simulink model "main"  (R2016b)
settings: Solver=VariableStepAuto  StartTime=0.0  StopTime=0.4  FixedStep=2e-4  RelTol=1e-3
values from neighbouring files (symbols this model uses):
  denGc = denGc{1}    [rigidBodyInit.m]
  numGc = numGc{1}    [rigidBodyInit.m]
  Ts = 1/fs    (= 0.0002)    [rigidBodyInit.m]
undefined symbols (not defined in the file or in its folder): denGp, denGpDis, numGp, numGpDis, TsN
libraries: model_controller x3, simulink x1
settings Model: Creator=Dai Luyao  LastModifiedBy=Dai Luyao

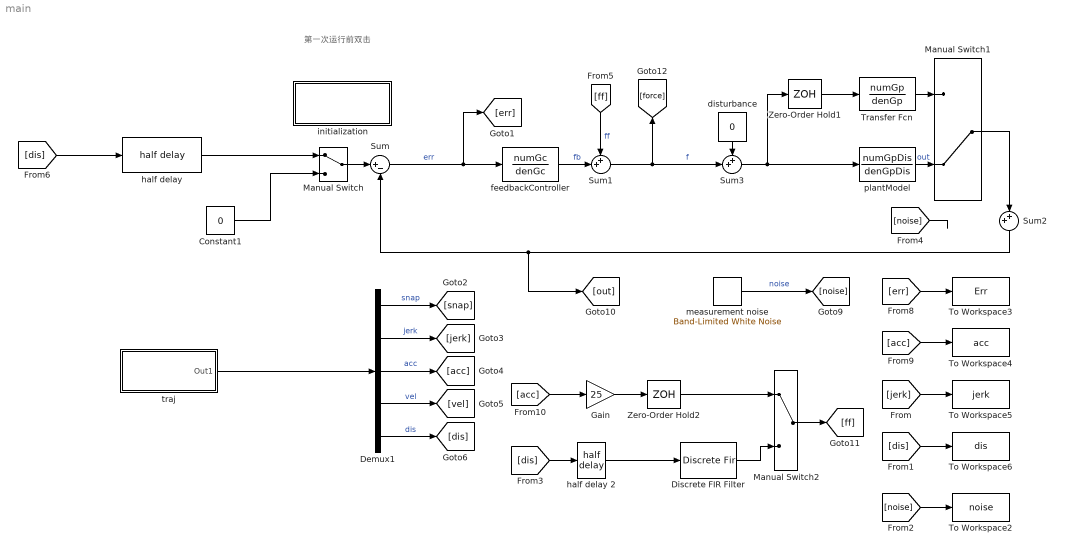
== system main ==
  note: 第一次运行前双击
  Constant1 : Constant  Value=0
  Demux1 : Demux  Outputs=5
  Discrete FIR Filter : DiscreteFir  Coefficients=denGpDis*6.25e8  SampleTime=Ts
  Gain : Gain  Gain=25
  Manual Switch : ManualSwitch
  Manual Switch1 : ManualSwitch  CurrentSetting=0
  Manual Switch2 : ManualSwitch
  Sum : Sum  Inputs=|+-
  Sum1 : Sum  Inputs=++|
  Sum2 : Sum  Inputs=++|
  Sum3 : Sum  Inputs=++|
  To Workspace2 : ToWorkspace  VariableName=noise  SaveFormat=Structure With Time  SampleTime=-1
  To Workspace3 : ToWorkspace  VariableName=Err  SaveFormat=Structure With Time  SampleTime=-1
  To Workspace4 : ToWorkspace  VariableName=acc  SaveFormat=Structure With Time  SampleTime=-1
  To Workspace5 : ToWorkspace  VariableName=jerk  SaveFormat=Structure With Time  SampleTime=-1
  To Workspace6 : ToWorkspace  VariableName=dis  SaveFormat=Structure With Time  SampleTime=-1
  Transfer Fcn : TransferFcn  Numerator=numGp  Denominator=denGp
  Zero-Order Hold1 : ZeroOrderHold  SampleTime=Ts
  Zero-Order Hold2 : ZeroOrderHold  SampleTime=Ts
  disturbance : Constant  Value=0
  feedbackController : DiscreteTransferFcn  Numerator=numGc  Denominator=denGc  SampleTime=Ts
  "half delay " : model_controller/Profile Generators/half delay 
  half delay 2 : model_controller/Profile Generators/half delay 
  initialization : Subsystem
      settings: OpenFcn=initiateSimulation;  MoveFcn=edit initiateSimulation;
  measurement noise : simulink/Sources/Band-Limited White Noise  Cov=noisePower  Ts=TsN  seed=[23341]
  plantModel : DiscreteTransferFcn  Numerator=numGpDis  Denominator=denGpDis  SampleTime=Ts
  traj : Subsystem  BlockChoice=4th order traj
      link override 3rd order traj: j=800  v=0.25  x=0.06  a=10
      link override 4th order traj: a=10  v=0.25
      settings: AttributesFormatString=%<BlockChoice>  TemplateBlock=model_controller/Profile Generators/traj  MemberBlocks=2nd order traj,3rd order traj,4th order traj,step,zero
  wires:
  Sum/1 -> feedbackController/1, [err]  "err"
  feedbackController/1 -> Sum1/2  "fb"
  Sum1/1 -> Sum3/2, [force]  "f"
  measurement noise/1 -> [noise]  "noise"
  Demux1/1 -> [snap]  "snap"
  Demux1/2 -> [jerk]  "jerk"
  Demux1/3 -> [acc]  "acc"
  Demux1/4 -> [vel]  "vel"
  Demux1/5 -> [dis]  "dis"
  [acc] -> To Workspace4/1
  [acc] -> Gain/1
  [jerk] -> To Workspace5/1
  traj/1(Out1) -> Demux1/1
  [ff] -> Sum1/1  "ff"
  [dis] -> To Workspace6/1
  [err] -> To Workspace3/1
  [noise] -> To Workspace2/1
  Manual Switch/1 -> Sum/1
  Constant1/1 -> Manual Switch/2
  disturbance/1 -> Sum3/1
  [dis] -> half delay 2/1
  half delay 2/1 -> Discrete FIR Filter/1
  Sum3/1 -> Zero-Order Hold1/1, plantModel/1
  Zero-Order Hold1/1 -> Transfer Fcn/1
  plantModel/1 -> Manual Switch1/2  "out"
  Transfer Fcn/1 -> Manual Switch1/1
  Manual Switch1/1 -> Sum2/2
  Discrete FIR Filter/1 -> Manual Switch2/2
  Manual Switch2/1 -> [ff]
  Sum2/1 -> Sum/2, [out]
  [dis] -> "half delay "/1
  "half delay "/1 -> Manual Switch/1
  Gain/1 -> Zero-Order Hold2/1
  Zero-Order Hold2/1 -> Manual Switch2/1
  [noise] -> ?

== system main/initialization ==

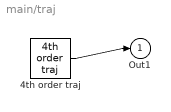
== system main/traj ==
  4th order traj : model_controller/Profile Generators/4th order traj  t0=0  x=0.06  v=0.25  a=10  j=800  d=64000  Ts=0
  Out1 : Outport
  wires:
  4th order traj/1 -> Out1/1
